simulink model "Task2"  (R2015b)
settings: Solver=VariableStepAuto  StartTime=0.0  StopTime=inf  RelTol=1e-3
settings Model: Creator=Irina_Novokhatskay  LastModifiedBy=User

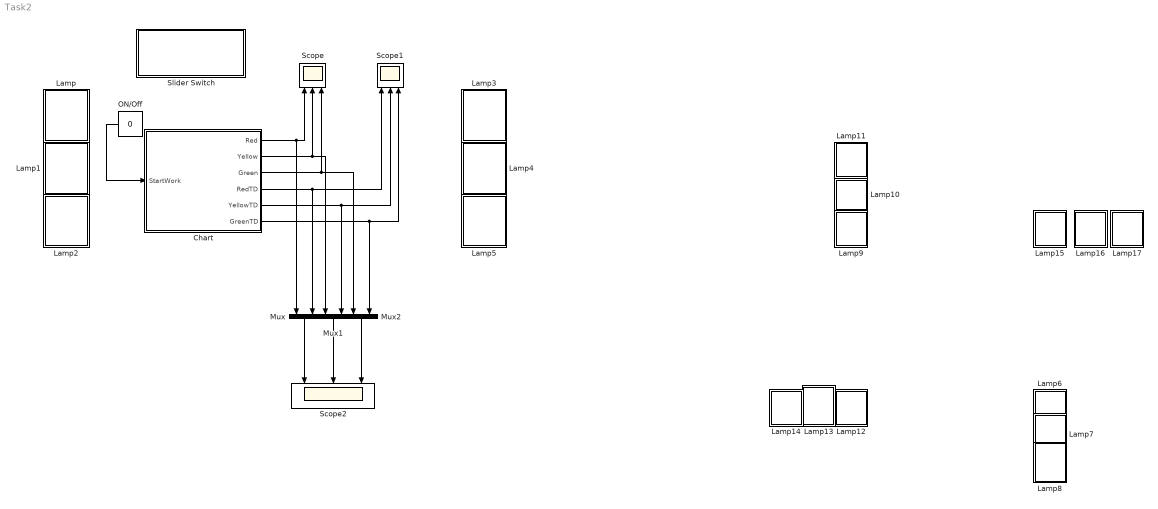
== system Task2 ==
  Chart : Stateflow chart  TreatAsAtomicUnit=on
  Lamp : Subsystem  DialogController=hmiCreateDDGDialog  IsWebBlock=on  mask(MWDashboardBlock){webBlockId=6a72cd25-3ace-4f89-9e8c-9b6b07c39fc1, webBlockType=lamp, ShowInLibBrowser=on, ShowInitialText=on, HMISrcModelName=Task2}
      mask prompts: webBlockType "WebBlock Type"; HMISrcModelName "Source Model"
      mask Help: helpview([docroot '/mapfiles/simulink.map'], 'hmi_lamp')
      mask Display:
      | if strcmp(get_param(bdroot(gcb),'BlockDiagramType'), 'library')
      |     image([(matlabroot) '/toolbox/simulink/hmi/icons/Lamp.png']);
      | end
  Lamp1 : Subsystem  DialogController=hmiCreateDDGDialog  IsWebBlock=on  mask(MWDashboardBlock){webBlockId=0b83c74a-5baa-4a76-abe6-b8eaac528e0c, webBlockType=lamp, ShowInLibBrowser=on, ShowInitialText=on, HMISrcModelName=Task2}
      mask prompts: webBlockType "WebBlock Type"; HMISrcModelName "Source Model"
      mask Help: helpview([docroot '/mapfiles/simulink.map'], 'hmi_lamp')
      mask Display:
      | if strcmp(get_param(bdroot(gcb),'BlockDiagramType'), 'library')
      |     image([(matlabroot) '/toolbox/simulink/hmi/icons/Lamp.png']);
      | end
  Lamp10 : Subsystem  DialogController=hmiCreateDDGDialog  IsWebBlock=on  mask(MWDashboardBlock){webBlockId=15f45251-5f67-42fd-ba7a-edb8e11b9a6a, webBlockType=lamp, ShowInLibBrowser=on, ShowInitialText=on, HMISrcModelName=Task2}
      mask prompts: webBlockType "WebBlock Type"; HMISrcModelName "Source Model"
      mask Help: helpview([docroot '/mapfiles/simulink.map'], 'hmi_lamp')
      mask Display:
      | if strcmp(get_param(bdroot(gcb),'BlockDiagramType'), 'library')
      |     image([(matlabroot) '/toolbox/simulink/hmi/icons/Lamp.png']);
      | end
  Lamp11 : Subsystem  DialogController=hmiCreateDDGDialog  IsWebBlock=on  mask(MWDashboardBlock){webBlockId=2de18072-848c-4ef7-bacd-9321842b3b74, webBlockType=lamp, ShowInLibBrowser=on, ShowInitialText=on, HMISrcModelName=Task2}
      mask prompts: webBlockType "WebBlock Type"; HMISrcModelName "Source Model"
      mask Help: helpview([docroot '/mapfiles/simulink.map'], 'hmi_lamp')
      mask Display:
      | if strcmp(get_param(bdroot(gcb),'BlockDiagramType'), 'library')
      |     image([(matlabroot) '/toolbox/simulink/hmi/icons/Lamp.png']);
      | end
  Lamp12 : Subsystem  DialogController=hmiCreateDDGDialog  IsWebBlock=on  mask(MWDashboardBlock){webBlockId=f8163705-30c2-478c-bfca-d909051ab481, webBlockType=lamp, ShowInLibBrowser=on, ShowInitialText=on, HMISrcModelName=Task2}
      mask prompts: webBlockType "WebBlock Type"; HMISrcModelName "Source Model"
      mask Help: helpview([docroot '/mapfiles/simulink.map'], 'hmi_lamp')
      mask Display:
      | if strcmp(get_param(bdroot(gcb),'BlockDiagramType'), 'library')
      |     image([(matlabroot) '/toolbox/simulink/hmi/icons/Lamp.png']);
      | end
  Lamp13 : Subsystem  DialogController=hmiCreateDDGDialog  IsWebBlock=on  mask(MWDashboardBlock){webBlockId=fc402684-b095-4abc-a5ce-f123ecd30ffe, webBlockType=lamp, ShowInLibBrowser=on, ShowInitialText=on, HMISrcModelName=Task2}
      mask prompts: webBlockType "WebBlock Type"; HMISrcModelName "Source Model"
      mask Help: helpview([docroot '/mapfiles/simulink.map'], 'hmi_lamp')
      mask Display:
      | if strcmp(get_param(bdroot(gcb),'BlockDiagramType'), 'library')
      |     image([(matlabroot) '/toolbox/simulink/hmi/icons/Lamp.png']);
      | end
  Lamp14 : Subsystem  DialogController=hmiCreateDDGDialog  IsWebBlock=on  mask(MWDashboardBlock){webBlockId=a8644dce-0fa4-41a3-b5a3-b7ded4881562, webBlockType=lamp, ShowInLibBrowser=on, ShowInitialText=on, HMISrcModelName=Task2}
      mask prompts: webBlockType "WebBlock Type"; HMISrcModelName "Source Model"
      mask Help: helpview([docroot '/mapfiles/simulink.map'], 'hmi_lamp')
      mask Display:
      | if strcmp(get_param(bdroot(gcb),'BlockDiagramType'), 'library')
      |     image([(matlabroot) '/toolbox/simulink/hmi/icons/Lamp.png']);
      | end
  Lamp15 : Subsystem  DialogController=hmiCreateDDGDialog  IsWebBlock=on  mask(MWDashboardBlock){webBlockId=7805cf90-d16b-4850-aef1-ca00daf5dcb3, webBlockType=lamp, ShowInLibBrowser=on, ShowInitialText=on, HMISrcModelName=Task2}
      mask prompts: webBlockType "WebBlock Type"; HMISrcModelName "Source Model"
      mask Help: helpview([docroot '/mapfiles/simulink.map'], 'hmi_lamp')
      mask Display:
      | if strcmp(get_param(bdroot(gcb),'BlockDiagramType'), 'library')
      |     image([(matlabroot) '/toolbox/simulink/hmi/icons/Lamp.png']);
      | end
  Lamp16 : Subsystem  DialogController=hmiCreateDDGDialog  IsWebBlock=on  mask(MWDashboardBlock){webBlockId=0230a9b6-90f6-42b8-9fba-191a9e515e07, webBlockType=lamp, ShowInLibBrowser=on, ShowInitialText=on, HMISrcModelName=Task2}
      mask prompts: webBlockType "WebBlock Type"; HMISrcModelName "Source Model"
      mask Help: helpview([docroot '/mapfiles/simulink.map'], 'hmi_lamp')
      mask Display:
      | if strcmp(get_param(bdroot(gcb),'BlockDiagramType'), 'library')
      |     image([(matlabroot) '/toolbox/simulink/hmi/icons/Lamp.png']);
      | end
  Lamp17 : Subsystem  DialogController=hmiCreateDDGDialog  IsWebBlock=on  mask(MWDashboardBlock){webBlockId=8a785a16-254f-44fb-8cfe-09d7cf8042f9, webBlockType=lamp, ShowInLibBrowser=on, ShowInitialText=on, HMISrcModelName=Task2}
      mask prompts: webBlockType "WebBlock Type"; HMISrcModelName "Source Model"
      mask Help: helpview([docroot '/mapfiles/simulink.map'], 'hmi_lamp')
      mask Display:
      | if strcmp(get_param(bdroot(gcb),'BlockDiagramType'), 'library')
      |     image([(matlabroot) '/toolbox/simulink/hmi/icons/Lamp.png']);
      | end
  Lamp2 : Subsystem  DialogController=hmiCreateDDGDialog  IsWebBlock=on  mask(MWDashboardBlock){webBlockId=e27a65a0-1e4d-4ed1-96a1-defa4afd1051, webBlockType=lamp, ShowInLibBrowser=on, ShowInitialText=on, HMISrcModelName=Task2}
      mask prompts: webBlockType "WebBlock Type"; HMISrcModelName "Source Model"
      mask Help: helpview([docroot '/mapfiles/simulink.map'], 'hmi_lamp')
      mask Display:
      | if strcmp(get_param(bdroot(gcb),'BlockDiagramType'), 'library')
      |     image([(matlabroot) '/toolbox/simulink/hmi/icons/Lamp.png']);
      | end
  Lamp3 : Subsystem  DialogController=hmiCreateDDGDialog  IsWebBlock=on  mask(MWDashboardBlock){webBlockId=9a19c506-71ae-4a57-994f-6279ef339d96, webBlockType=lamp, ShowInLibBrowser=on, ShowInitialText=on, HMISrcModelName=Task2}
      mask prompts: webBlockType "WebBlock Type"; HMISrcModelName "Source Model"
      mask Help: helpview([docroot '/mapfiles/simulink.map'], 'hmi_lamp')
      mask Display:
      | if strcmp(get_param(bdroot(gcb),'BlockDiagramType'), 'library')
      |     image([(matlabroot) '/toolbox/simulink/hmi/icons/Lamp.png']);
      | end
  Lamp4 : Subsystem  DialogController=hmiCreateDDGDialog  IsWebBlock=on  mask(MWDashboardBlock){webBlockId=34e4b4fc-f0f9-4732-bebf-acbc3324067c, webBlockType=lamp, ShowInLibBrowser=on, ShowInitialText=on, HMISrcModelName=Task2}
      mask prompts: webBlockType "WebBlock Type"; HMISrcModelName "Source Model"
      mask Help: helpview([docroot '/mapfiles/simulink.map'], 'hmi_lamp')
      mask Display:
      | if strcmp(get_param(bdroot(gcb),'BlockDiagramType'), 'library')
      |     image([(matlabroot) '/toolbox/simulink/hmi/icons/Lamp.png']);
      | end
  Lamp5 : Subsystem  DialogController=hmiCreateDDGDialog  IsWebBlock=on  mask(MWDashboardBlock){webBlockId=46939de4-5fc6-4d9b-a5f7-006a554046a3, webBlockType=lamp, ShowInLibBrowser=on, ShowInitialText=on, HMISrcModelName=Task2}
      mask prompts: webBlockType "WebBlock Type"; HMISrcModelName "Source Model"
      mask Help: helpview([docroot '/mapfiles/simulink.map'], 'hmi_lamp')
      mask Display:
      | if strcmp(get_param(bdroot(gcb),'BlockDiagramType'), 'library')
      |     image([(matlabroot) '/toolbox/simulink/hmi/icons/Lamp.png']);
      | end
  Lamp6 : Subsystem  DialogController=hmiCreateDDGDialog  IsWebBlock=on  mask(MWDashboardBlock){webBlockId=41663ddb-bc88-46f9-83ac-f1e7484bb24e, webBlockType=lamp, ShowInLibBrowser=on, ShowInitialText=on, HMISrcModelName=Task2}
      mask prompts: webBlockType "WebBlock Type"; HMISrcModelName "Source Model"
      mask Help: helpview([docroot '/mapfiles/simulink.map'], 'hmi_lamp')
      mask Display:
      | if strcmp(get_param(bdroot(gcb),'BlockDiagramType'), 'library')
      |     image([(matlabroot) '/toolbox/simulink/hmi/icons/Lamp.png']);
      | end
  Lamp7 : Subsystem  DialogController=hmiCreateDDGDialog  IsWebBlock=on  mask(MWDashboardBlock){webBlockId=3a8707aa-c691-48fb-b5ca-e343ac96153c, webBlockType=lamp, ShowInLibBrowser=on, ShowInitialText=on, HMISrcModelName=Task2}
      mask prompts: webBlockType "WebBlock Type"; HMISrcModelName "Source Model"
      mask Help: helpview([docroot '/mapfiles/simulink.map'], 'hmi_lamp')
      mask Display:
      | if strcmp(get_param(bdroot(gcb),'BlockDiagramType'), 'library')
      |     image([(matlabroot) '/toolbox/simulink/hmi/icons/Lamp.png']);
      | end
  Lamp8 : Subsystem  DialogController=hmiCreateDDGDialog  IsWebBlock=on  mask(MWDashboardBlock){webBlockId=01bae4a3-615c-4b87-9642-9742c6fff1f3, webBlockType=lamp, ShowInLibBrowser=on, ShowInitialText=on, HMISrcModelName=Task2}
      mask prompts: webBlockType "WebBlock Type"; HMISrcModelName "Source Model"
      mask Help: helpview([docroot '/mapfiles/simulink.map'], 'hmi_lamp')
      mask Display:
      | if strcmp(get_param(bdroot(gcb),'BlockDiagramType'), 'library')
      |     image([(matlabroot) '/toolbox/simulink/hmi/icons/Lamp.png']);
      | end
  Lamp9 : Subsystem  DialogController=hmiCreateDDGDialog  IsWebBlock=on  mask(MWDashboardBlock){webBlockId=79ace46e-a0a5-4d52-b8a3-0b07a0b6810c, webBlockType=lamp, ShowInLibBrowser=on, ShowInitialText=on, HMISrcModelName=Task2}
      mask prompts: webBlockType "WebBlock Type"; HMISrcModelName "Source Model"
      mask Help: helpview([docroot '/mapfiles/simulink.map'], 'hmi_lamp')
      mask Display:
      | if strcmp(get_param(bdroot(gcb),'BlockDiagramType'), 'library')
      |     image([(matlabroot) '/toolbox/simulink/hmi/icons/Lamp.png']);
      | end
  Mux : Mux  Inputs=2
  Mux1 : Mux  Inputs=2
  Mux2 : Mux  Inputs=2
  ON/Off : Constant  Value=0  OutDataTypeStr=boolean
  Scope : Scope  NumInputPorts=3
  Scope1 : Scope  NumInputPorts=3
  Scope2 : Scope  NumInputPorts=3
  Slider Switch : Subsystem  DialogController=hmiCreateDDGDialog  IsWebBlock=on  mask(MWDashboardBlock){webBlockId=e1889411-aa88-4b88-80a0-3b85c20c65d0, webBlockType=sliderswitch, ShowInLibBrowser=on, ShowInitialText=on, HMISrcModelName=Task2}
      mask prompts: webBlockId "WebBlock Id"; webBlockType "WebBlock Type"; HMISrcModelName "Source Model"
      mask Help: helpview([docroot '/mapfiles/simulink.map'], 'hmi_slider_switch')
      mask Display:
      | if strcmp(get_param(bdroot(gcb),'BlockDiagramType'), 'library')
      |     image([(matlabroot) '/toolbox/simulink/hmi/icons/SliderSwitch.png']);
      | end
  wires:
  Chart/1(Red) -> Scope/1, Mux/1
  Chart/2(Yellow) -> Mux1/1, Scope/2
  Chart/3(Green) -> Scope/3, Mux2/1
  Chart/4(RedTD) -> Scope1/1, Mux/2
  Chart/5(YellowTD) -> Scope1/2, Mux1/2
  Chart/6(GreenTD) -> Scope1/3, Mux2/2
  ON/Off/1 -> Chart/1(StartWork)
  Mux/1 -> Scope2/1
  Mux1/1 -> Scope2/2
  Mux2/1 -> Scope2/3

== system Task2/Lamp ==

== system Task2/Lamp1 ==

== system Task2/Lamp10 ==

== system Task2/Lamp11 ==

== system Task2/Lamp12 ==

== system Task2/Lamp13 ==

== system Task2/Lamp14 ==

== system Task2/Lamp15 ==

== system Task2/Lamp16 ==

== system Task2/Lamp17 ==

== system Task2/Lamp2 ==

== system Task2/Lamp3 ==

== system Task2/Lamp4 ==

== system Task2/Lamp5 ==

== system Task2/Lamp6 ==

== system Task2/Lamp7 ==

== system Task2/Lamp8 ==

== system Task2/Lamp9 ==

== system Task2/Slider Switch ==

== stateflow chart Task2/Chart ==
  state Controler
    state TrafickLiteLogic [parallel]
      settings: executionOrder=1
      state YellowBlink1
        entry: Red=0;
        Yellow=0;
        Green=0;
      state YellowBlink
        entry: Red=0;
        Yellow=1;
        Green=0;
      state Red
        entry: Red=1;
        Yellow = 0;
        Green=0;
        state RedAndYellow
          entry:
          Red =1;
          Yellow=1;
          Green = 0;
          Block=true;
        state Delay
          entry:
          Turn=false;
        (default) -> Delay
        Delay -> RedAndYellow : [Turn]
      state Yellow
        entry:
        Red=0;
        Yellow=1;
        Green=0;
      state GreenBlink1
        entry:
        Red=0;
        Yellow=0;
        Green=0;
        GBL = GBL + 1;
      state GreenBlink
        entry:
        Red=0;
        Yellow=0;
        Green=1;
      state Green
        entry:
        Red=0;
        Yellow=0;
        Green=1;
        GBL = 0;
      (default) -> YellowBlink
      YellowBlink -> YellowBlink1 [order 1] : [after(1,sec) && ~StartWork]
      YellowBlink1 -> YellowBlink : after(1,sec)
      YellowBlink -> RedAndYellow [order 2] : [StartWork]
      RedAndYellow -> Green : after(5,sec)
      Yellow -> Red : after(5,sec)
      GreenBlink -> Yellow [order 2] : [GBL==3]
      GreenBlink -> GreenBlink1 [order 1] : [after(1,sec) &&GBL~=3 ]
      GreenBlink1 -> GreenBlink : after(1,sec)
      Green -> GreenBlink : after(40,sec)
    state TrafickLiteLogic1 [parallel]
      settings: executionOrder=2
      state YellowBlink1TD
        entry: RedTD=0;
        YellowTD=0;
        GreenTD=0;
      state YellowBlinkTD
        entry: RedTD=0;
        YellowTD=1;
        GreenTD=0;
      state RedTD
        entry: RedTD=1;
        YellowTD = 0;
        GreenTD=0;
        state RedAndYellowTD
          entry:
          RedTD =1;
          YellowTD=1;
          GreenTD = 0;
          Block=true;
        state DelayTD
          entry:
          Turn=true;
        DelayTD -> RedAndYellowTD : [~Turn]
        (default) -> DelayTD
      state YellowTD
        entry:
        RedTD=0;
        YellowTD=1;
        GreenTD=0;
      state GreenBlink1TD
        entry:
        RedTD=0;
        YellowTD=0;
        GreenTD=0;
        GBLTD = GBLTD + 1;
      state GreenBlinkTD
        entry:
        RedTD=0;
        YellowTD=0;
        GreenTD=1;
      state GreenTD
        entry:
        RedTD=0;
        YellowTD=0;
        GreenTD=1;
        GBLTD = 0;
      (default) -> YellowBlinkTD
      YellowBlinkTD -> YellowBlink1TD [order 1] : [after(1,sec) && ~StartWork]
      YellowBlink1TD -> YellowBlinkTD : after(1,sec)
      YellowBlinkTD -> RedTD [order 2] : [StartWork]
      RedAndYellowTD -> GreenTD : after(5,sec)
      YellowTD -> RedTD : after(5,sec)
      GreenBlinkTD -> YellowTD [order 2] : [GBLTD==3]
      GreenBlinkTD -> GreenBlink1TD [order 1] : [after(1,sec) &&GBLTD~=3 ]
      GreenBlink1TD -> GreenBlinkTD : after(1,sec)
      GreenTD -> GreenBlinkTD : after(40,sec)
    state TurnLogic [parallel]
      settings: executionOrder=3
      state Wait
      (default) -> Wait
  data: Red output; Yellow output; Green output; GBL local; RedTD output; YellowTD output; GreenTD output; GBLTD local; Turn local boolean; StartWork input boolean; Block local boolean
